simulink model "Simulink_Practica_1"  (R2022a)
settings: Solver=VariableStepAuto  StartTime=0  StopTime=10.0  MaxStep=0.001  RelTol=1e-3
values from neighbouring files (symbols this model uses):
  g = 9.81    [Matlab_Practica_1.m]
  L1 = 0.3    [Matlab_Practica_1.m]
  L2 = 0.25    [Matlab_Practica_1.m]
  m1 = 0.2    [Matlab_Practica_1.m]
  m2 = 0.1    [Matlab_Practica_1.m]
settings Model: Creator=PC  LastModifiedBy=PC

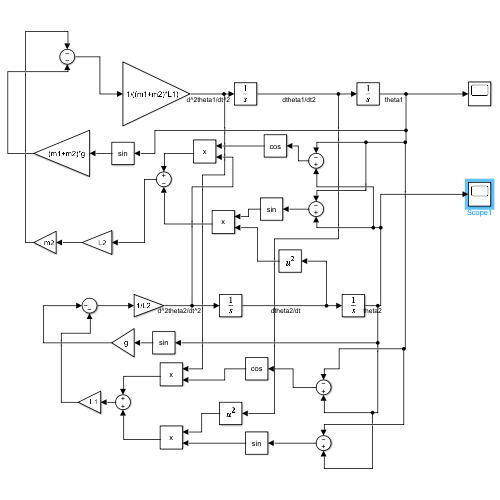
[thumbnail: Simulink's stored preview of the top-level diagram]
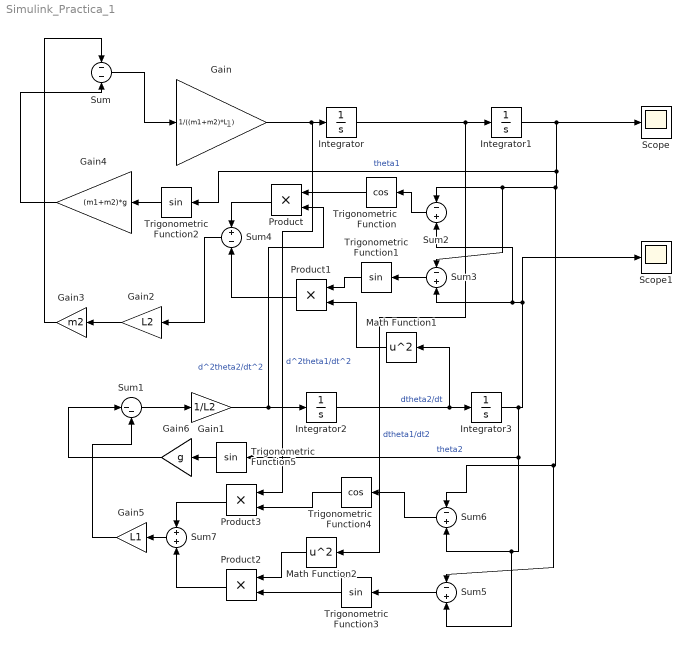
== system Simulink_Practica_1 ==
  note: 1
  Gain : Gain  Gain=1/((m1+m2)*L1)
  Gain1 : Gain  Gain=1/L2
  Gain2 : Gain  Gain=L2
  Gain3 : Gain  Gain=m2
  Gain4 : Gain  Gain=(m1+m2)*g
  Gain5 : Gain  Gain=L1
  Gain6 : Gain  Gain=g
  Integrator : Integrator
  Integrator1 : Integrator
  Integrator2 : Integrator
  Integrator3 : Integrator  InitialCondition=(35*pi)/180
  Math Function1 : Math  Operator=square
  Math Function2 : Math  Operator=square
  Product{,1..3} (4 alike) : Product
  Scope : Scope
  Scope1 : Scope
  Sum : Sum  Inputs=--
  Sum1 : Sum  Inputs=|--
  Sum{2..3,5..6} (4 alike) : Sum  Inputs=-+
  Sum4 : Sum  Inputs=+-
  Sum7 : Sum
  Trigonometric Function : Trigonometry  Operator=cos
  Trigonometric Function{1..3,5} (4 alike) : Trigonometry
  Trigonometric Function4 : Trigonometry  Operator=cos
  wires:
  Integrator/1 -> Math Function2/1, Integrator1/1  "dtheta1/dt2"
  Integrator2/1 -> Math Function1/1, Integrator3/1  "dtheta2/dt"
  Gain/1 -> Product3/1, Integrator/1  "d^2theta1/dt^2"
  Gain1/1 -> Product/2, Integrator2/1  "d^2theta2/dt^2"
  Sum/1 -> Gain/1
  Sum1/1 -> Gain1/1
  Integrator1/1 -> Sum5/1, Sum6/1, Sum2/1, Sum3/1, Trigonometric Function2/1, Scope/1  "theta1"
  Integrator3/1 -> Trigonometric Function5/1, Sum5/2, Sum6/2, Scope1/1, Sum3/2, Sum2/2  "theta2"
  Sum2/1 -> Trigonometric Function/1
  Sum3/1 -> Trigonometric Function1/1
  Trigonometric Function/1 -> Product/1
  Product/1 -> Sum4/1
  Trigonometric Function1/1 -> Product1/1
  Product1/1 -> Sum4/2
  Sum4/1 -> Gain2/1
  Trigonometric Function2/1 -> Gain4/1
  Gain3/1 -> Sum/1
  Sum6/1 -> Trigonometric Function4/1
  Sum5/1 -> Trigonometric Function3/1
  Trigonometric Function3/1 -> Product2/2
  Trigonometric Function4/1 -> Product3/2
  Product2/1 -> Sum7/2
  Product3/1 -> Sum7/1
  Sum7/1 -> Gain5/1
  Gain5/1 -> Sum1/2
  Trigonometric Function5/1 -> Gain6/1
  Gain6/1 -> Sum1/1
  Math Function2/1 -> Product2/1
  Math Function1/1 -> Product1/2
  Gain2/1 -> Gain3/1
  Gain4/1 -> Sum/2
